simulink model "erfan_1"  (R2018b)
settings: Solver=VariableStepAuto  StartTime=0.0  StopTime=10.0  RelTol=1e-3
values from neighbouring files (symbols this model uses):
  Ct = double( subs( Ct) )    [main_sys.m]    (also in main_sys_klm.m; main_tf_10.m; main_tf_11.m; main_tf_12.m)
  K = P*C'/(C*P*C' + R)    [KALMAN.m]    (also in main_tf_9.m = lqi(sys_lq,Q,R))
  sys_sys = ss(A,B,C,D)    [main_sys.m]    (also in main_sys_klm.m; main_tf_10.m; main_tf_11.m; main_tf_12.m = ss(A_sys,B_sys,C_sys_mod,D_sys_mod))
settings Model: Creator=eshojaei  LastModifiedBy=eshojaei

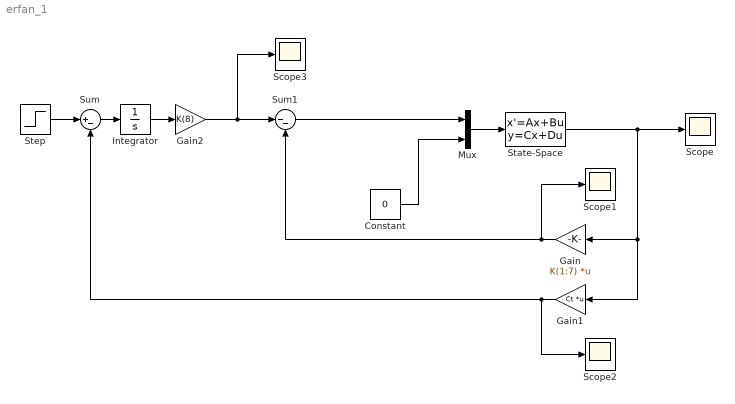
== system erfan_1 ==
  Constant : Constant  Value=0
  Gain : Gain  Gain=K(1:7)  Multiplication=Matrix(K*u)
  Gain1 : Gain  Gain=Ct  Multiplication=Matrix(K*u)
  Gain2 : Gain  Gain=K(8)
  Integrator : Integrator
  Mux : Mux  Inputs=2
  Scope{,1..3} (4 alike) : Scope
  State-Space : StateSpace  A=sys_sys.A  B=sys_sys.B  C=sys_sys.C  D=sys_sys.D  InitialCondition=0
  Step : Step  Time=.1  After=5  SampleTime=0
  Sum : Sum  Inputs=|+-
  Sum1 : Sum  Inputs=|--
  wires:
  Mux/1 -> State-Space/1
  State-Space/1 -> Gain1/1, Gain/1, Scope/1
  Constant/1 -> Mux/2
  Gain/1 -> Sum1/2, Scope1/1
  Step/1 -> Sum/1
  Gain1/1 -> Scope2/1, Sum/2
  Sum/1 -> Integrator/1
  Integrator/1 -> Gain2/1
  Gain2/1 -> Sum1/1, Scope3/1
  Sum1/1 -> Mux/1
